simulink model "PC_MSFS_STATION"  (R2021b)
settings: Solver=FixedStepAuto  StartTime=0.0  StopTime=600  FixedStep=0.03  RelTol=1e-3
undefined symbols (not defined in the file): DiscIntNeverNeededParam, MODEL, MODEL_INI
libraries: SimConnectToolbox x9, simulink x4
(part 2 of 2)

== matlab function PC_MSFS_STATION/SYSTEM/UNICYCLE MODEL ==
  data: STATE input; STATE_DERIVATIVE output; MODEL_IN input; MODEL output Bus: MODEL_Bus
function [STATE_DERIVATIVE,MODEL] = SO_UNICYCLE_MODEL(STATE, MODEL_IN)
% COPY MODEL BUS
MODEL = MODEL_IN;
%--------------------------------------------------------------------------
% SO UNICYCLE PARAMETERS
%--------------------------------------------------------------------------
dist_p = MODEL.PARAM.DISP_P;
flight_status = MODEL.PARAM.FLIGHT_STATUS;
switch_flag = MODEL.PARAM.SWTCH_FLAG;
%--------------------------------------------------------------------------
% EVALUATE FLIGHT STATUS
%--------------------------------------------------------------------------
if flight_status == 0
    % INITIALIZATION
    theta_long = MODEL.INPUT.LONGITUDE;
    phi_lat = MODEL.INPUT.LATITUDE;
    altitude = MODEL.INPUT.ALTITUDE;
    rho = altitude + 20.902e6;
    % Displaced Point Dynamics Y = {y1, y2, vy1, vy2}
    y1 = rho*cos(phi_lat)*cos(theta_long);
    y2 = rho*cos(phi_lat)*sin(theta_long);
    vy1 = 0;
    vy2 = 0;
    % Center of Mass Dynamics X = {x1, x2, s, theta, omega}
    s = 0;
    theta = 0;
    omega = 0;
    x1 = y1 - dist_p*cos(theta);
    x2 = y2 - dist_p*sin(theta);
    switch_flag = 1;
% elseif flight_status == 1
%     % TAKE OFF
%     theta_long = MODEL.INPUT.LONGITUDE;
%     phi_lat = MODEL.INPUT.LATITUDE;
%     altitude = MODEL.INPUT.ALTITUDE;
%     rho = altitude + 20.902e6;
%     % Displaced Point Dynamics Y = {y1, y2, vy1, vy2}
%     y1 = rho*cos(phi_lat)*cos(theta_long);
%     y2 = rho*cos(phi_lat)*sin(theta_long);
%     vy1 = 0;
%     vy2 = 0;
%     % Center of Mass Dynamics X = {x1, x2, s, theta, omega}
%     s = 0;
%     theta = 0;
%     omega = 0;
%     x1 = y1 - dist_p*cos(theta);
%     x2 = y2 - dist_p*sin(theta);
else
    % ON FLIGHT
    %--------------------------------------------------------------------------
    % STATE VARIABLES
    %--------------------------------------------------------------------------
    % Displaced Point Dynamics Y = {y1, y2, vy1, vy2}
    y1 = STATE(1);
    y2 = STATE(2);
    vy1 = STATE(3);
    vy2 = STATE(4);
    % Center of Mass Dynamics X = {x1, x2, s, theta, omega}
    s = STATE(5);
    theta = STATE(6);
    omega = STATE(7);
    x1 = y1 - dist_p*cos(theta);
    x2 = y2 - dist_p*sin(theta);

end

%--------------------------------------------------------------------------
% INPUTS
%--------------------------------------------------------------------------
tau1 = MODEL.INPUT.TAU1;
tau2 = MODEL.INPUT.TAU2;
%--------------------------------------------------------------------------
% STATE EQUATIONS
%--------------------------------------------------------------------------
y1dot = vy1;
y2dot = vy2;
y1ddot = tau1;
y2ddot = tau2;
sdot = -omega^2*dist_p + tau1*cos(theta) + tau2*sin(theta);
thetadot = omega;
omegadot = 1/dist_p*(omega*s - tau1*sin(theta) + tau2*cos(theta));
%--------------------------------------------------------------------------
% STATE DERIVATIVES
%--------------------------------------------------------------------------
% if (flight_status > 0)&&(switch_flag == 1)
%     STATE_DERIVATIVE = [1; 1; 0; 0; 0; 0; 0];
%     switch_flag = 0;
% else
%     STATE_DERIVATIVE = [y1dot; y2dot; y1ddot; y2ddot; sdot; thetadot; omegadot];
% end

STATE_DERIVATIVE = [y1dot; y2dot; y1ddot; y2ddot; sdot; thetadot; omegadot];

%%%%%%%%%%%%%%%%%%%%%%%%%%%%%%%%%%%%%%%%%%%%%%%%%%%%%%%%%%%%%%%%%%%%%%%%%%%
% OUTPUT BUS
%%%%%%%%%%%%%%%%%%%%%%%%%%%%%%%%%%%%%%%%%%%%%%%%%%%%%%%%%%%%%%%%%%%%%%%%%%%
MODEL.STATE = [y1 ; y2 ; vy1 ; vy2 ; s ; theta ; omega];
MODEL.OUTPUT.X1 = x1;
MODEL.OUTPUT.X2 = x2;
MODEL.OUTPUT.X = sqrt(x1^2 + x2^2);
MODEL.OUTPUT.Y = sqrt(y1^2 + y2^2);
MODEL.PARAM.SWTCH_FLAG = switch_flag;
% TBD: SPHERICAL COORDINATES
% MODEL.OUTPUT.ALTITUDE = 0;
% MODEL.OUTPUT.LATITUDE = 0;
% MODEL.OUTPUT.LONGITUDE = 0;
return
